simulink model "DroneModelV2"  (R2024a)
settings: Solver=VariableStepAuto  StartTime=0.0  StopTime=7  RelTol=1e-3
values from neighbouring files (symbols this model uses):
  drag_co = torque_Nm / no_rot^2    (= 9.75332775919e-12)    [QuadcopterAttributes.m]
  g = 9.81    [StateSpace.m]
  KV_rating = 2800    [QuadcopterAttributes.m]
  lift_co = thrust_N / no_rot^2    (= 5.88883004597e-10)    [QuadcopterAttributes.m]
  m = 0.5    [StateSpace.m]
  r = 0.25    [StateSpace.m]
undefined symbols (not defined in the file or in its folder): I_p
libraries: simulink x2, shared6dof x1
settings Model: Creator=Henrik  LastModifiedBy=Henrik

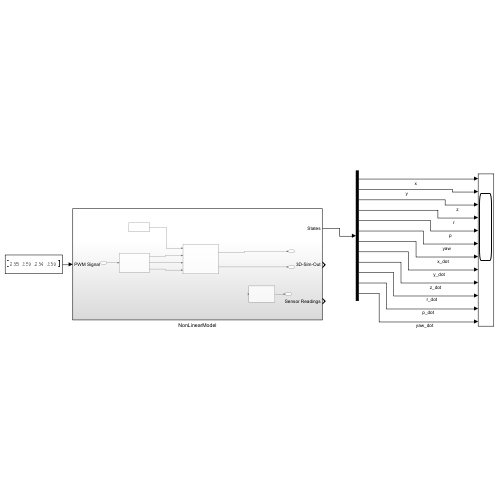
[thumbnail: Simulink's stored preview of the top-level diagram]
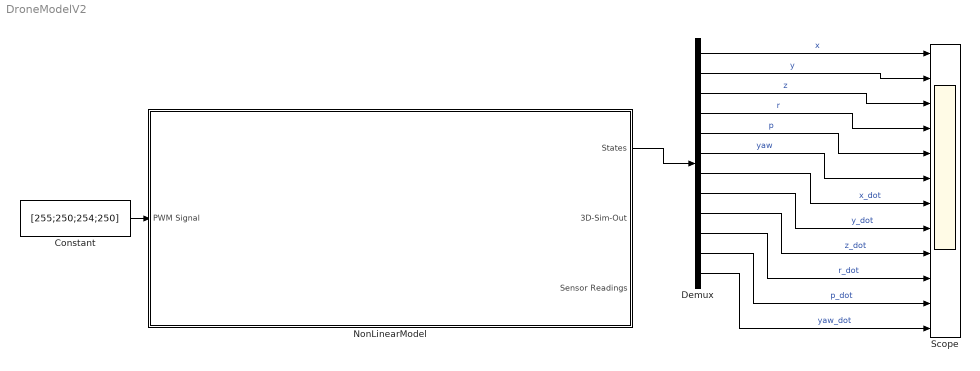
== system DroneModelV2 ==
  Constant : Constant  Value=[255;250;254;250]
  Demux : Demux  Outputs=12
  NonLinearModel : Subsystem
  Scope : Scope  NumInputPorts=12
  wires:
  Constant/1 -> NonLinearModel/1(PWM Signal)
  NonLinearModel/1(States) -> Demux/1
  Demux/1 -> Scope/1  "x"
  Demux/2 -> Scope/2  "y"
  Demux/3 -> Scope/3  "z"
  Demux/4 -> Scope/4  "r"
  Demux/5 -> Scope/5  "p"
  Demux/6 -> Scope/6  "yaw"
  Demux/7 -> Scope/7  "x_dot"
  Demux/8 -> Scope/8  "y_dot"
  Demux/9 -> Scope/9  "z_dot"
  Demux/10 -> Scope/10  "r_dot"
  Demux/11 -> Scope/11  "p_dot"
  Demux/12 -> Scope/12  "yaw_dot"

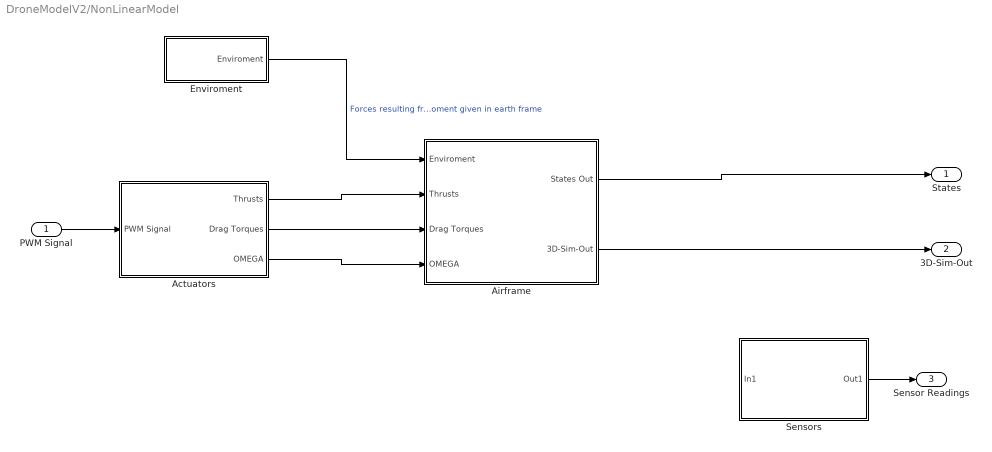
== system DroneModelV2/NonLinearModel ==
  PWM Signal : Inport
  Actuators : Subsystem
  Airframe : Subsystem
  Enviroment : Subsystem
  Sensors : Subsystem
  States : Outport
  3D-Sim-Out : Outport  Port=2
  Sensor Readings : Outport  Port=3
  wires:
  PWM Signal/1 -> Actuators/1(PWM Signal)
  Airframe/1(States Out) -> States/1
  Enviroment/1(Enviroment) -> Airframe/1(Enviroment)  "Forces resulting from enviroment given in earth frame"
  Actuators/1(Thrusts) -> Airframe/2(Thrusts)
  Airframe/2(3D-Sim-Out) -> 3D-Sim-Out/1
  Actuators/2(Drag Torques) -> Airframe/3(Drag Torques)
  Actuators/3(OMEGA) -> Airframe/4(OMEGA)
  Sensors/1(Out1) -> Sensor Readings/1

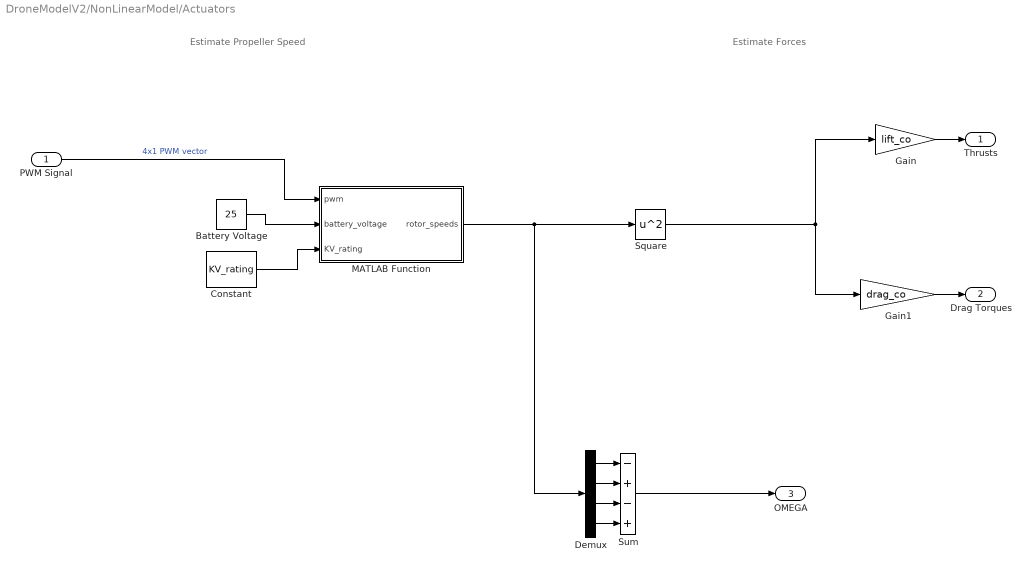
== system DroneModelV2/NonLinearModel/Actuators ==
  note: Estimate Forces
  note: Estimate Propeller Speed
  PWM Signal : Inport
  Battery Voltage : Constant  Value=25
  Constant : Constant  Value=KV_rating
  Demux : Demux
  Gain : Gain  Gain=lift_co
  Gain1 : Gain  Gain=drag_co
  MATLAB Function : MATLAB Function  TreatAsAtomicUnit=on
  Square : Math  Operator=square
  Sum : Sum  Inputs=-+-+
  Thrusts : Outport
  Drag Torques : Outport  Port=2
  OMEGA : Outport  Port=3
  wires:
  Constant/1 -> MATLAB Function/3(KV_rating)
  Battery Voltage/1 -> MATLAB Function/2(battery_voltage)
  PWM Signal/1 -> MATLAB Function/1(pwm)  "4x1 PWM vector"
  MATLAB Function/1(rotor_speeds) -> Square/1, Demux/1
  Gain/1 -> Thrusts/1
  Square/1 -> Gain/1, Gain1/1
  Gain1/1 -> Drag Torques/1
  Demux/1 -> Sum/1
  Demux/2 -> Sum/2
  Demux/3 -> Sum/3
  Demux/4 -> Sum/4
  Sum/1 -> OMEGA/1

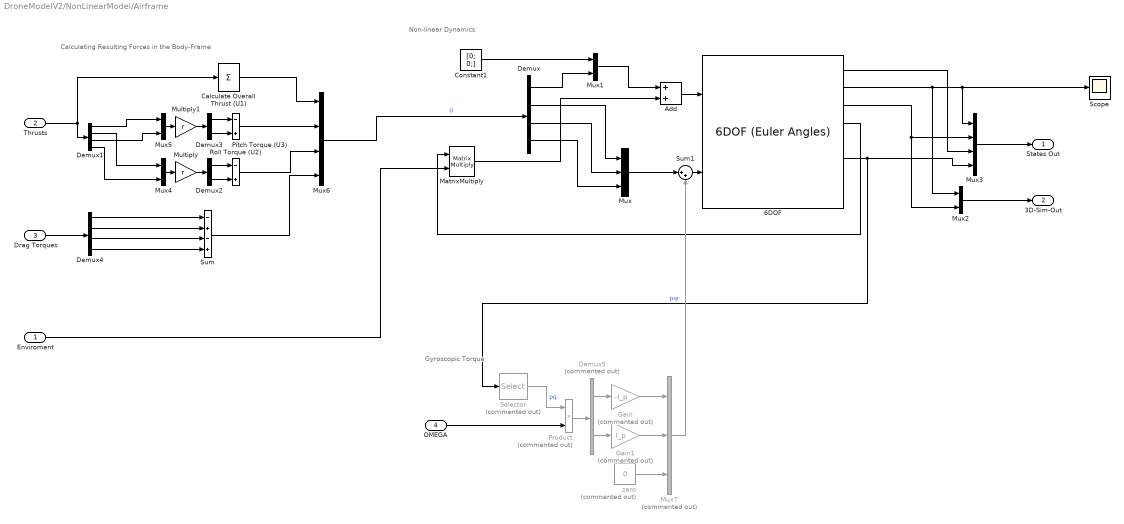
== system DroneModelV2/NonLinearModel/Airframe ==
  note: Gyroscopic Torque
  note: Non-linear Dynamics
  note: Calculating Resulting Forces in the Body-Frame
  Enviroment : Inport
  Thrusts : Inport  Port=2
  Drag Torques : Inport  Port=3
  OMEGA : Inport  Port=4
  "6DOF " : shared6dof/6DOF (Euler Angles)  units=Metric (MKS)  mtype=Fixed  rep=Quaternion  xme_0=[0 0 0]  Vm_0=[0 0 0]  eul_0=[0 0 0]  pm_0=[0 0 0]  mass_0=m  mass_e=0.5  mass_f=2.0  inertia=Inertia_Mat  inertia_e=eye(3)  inertia_f=2*eye(3)  k_quat=1.0  vre_flag=on  abi_flag=off  aMode=0  xme_statename=''  Vm_statename=''  eul_statename=''  quat_statename=''  pm_statename=''  mass_statename=''
      settings: LibrarySourceBlock=aerolib6dof2/6DOF (Quaternion)
  Add : Sum
  "Calculate Overall Thrust (U1) " : Sum  Inputs=+
  Constant1 : Constant  Value=[0; 0;]
  Demux : Demux
  Demux1 : Demux
  Demux2 : Demux  Outputs=2
  Demux3 : Demux  Outputs=2
  Demux4 : Demux
  Demux5 : Demux  Commented=on  Outputs=2
  Gain : Gain  Commented=on  Gain=-I_p
  Gain1 : Gain  Commented=on  Gain=I_p
  MatrixMultiply : Product  Multiplication=Matrix(*)
  Multiply : Gain  Gain=r
  Multiply1 : Gain  Gain=r
  Mux : Mux  Inputs=3
  Mux{1..2,4..5} (4 alike) : Mux  Inputs=2
  Mux3 : Mux
  Mux6 : Mux
  Mux7 : Mux  Commented=on  Inputs=3
  Pitch Torque (U3) : Sum  Inputs=-+
  Product : Product  Commented=on
  Roll Torque (U2) : Sum  Inputs=-+
  Scope : Scope
  Selector : Selector  Commented=on  InputPortWidth=3  IndexOptions=Index vector (dialog)  Indices=[1 2]  OutputSizes=1
  Sum : Sum  Inputs=-+-+
  Sum1 : Sum  Inputs=|++
  zero : Constant  Commented=on  Value=0
  States Out : Outport
  3D-Sim-Out : Outport  Port=2
  wires:
  Demux/2 -> Mux/1
  Demux/3 -> Mux/2
  Demux/4 -> Mux/3
  Enviroment/1 -> MatrixMultiply/2
  "6DOF "/4 -> MatrixMultiply/1
  Add/1 -> "6DOF "/1
  MatrixMultiply/1 -> Add/2
  "6DOF "/2 -> Mux2/1, Mux3/1, Scope/1
  Demux/1 -> Mux1/2
  Constant1/1 -> Mux1/1
  Mux1/1 -> Add/1
  Mux2/1 -> 3D-Sim-Out/1
  "6DOF "/3 -> Mux3/2, Mux2/2
  "6DOF "/1 -> Mux3/3
  "6DOF "/6 -> Mux3/4, Selector/1  "pqr"
  Mux3/1 -> States Out/1
  Thrusts/1 -> "Calculate Overall Thrust (U1) "/1, Demux1/1
  Demux1/4 -> Mux4/2
  Demux1/2 -> Mux4/1
  Mux4/1 -> Multiply/1
  Multiply/1 -> Demux2/1
  Demux2/1 -> Roll Torque (U2)/1
  Demux2/2 -> Roll Torque (U2)/2
  Mux5/1 -> Multiply1/1
  Demux1/1 -> Mux5/1
  Multiply1/1 -> Demux3/1
  Demux3/2 -> Pitch Torque (U3)/2
  Demux3/1 -> Pitch Torque (U3)/1
  Demux1/3 -> Mux5/2
  "Calculate Overall Thrust (U1) "/1 -> Mux6/1
  Pitch Torque (U3)/1 -> Mux6/2
  Roll Torque (U2)/1 -> Mux6/3
  Mux6/1 -> Demux/1  "U"
  Drag Torques/1 -> Demux4/1
  Demux4/3 -> Sum/3
  Demux4/4 -> Sum/4
  Demux4/1 -> Sum/1
  Demux4/2 -> Sum/2
  Sum/1 -> Mux6/4
  OMEGA/1 -> Product/2
  Selector/1 -> Product/1  "pq"
  Product/1 -> Demux5/1
  Demux5/1 -> Gain/1
  Demux5/2 -> Gain1/1
  Gain/1 -> Mux7/1
  Gain1/1 -> Mux7/2
  zero/1 -> Mux7/3
  Mux/1 -> Sum1/1
  Mux7/1 -> Sum1/2
  Sum1/1 -> "6DOF "/2

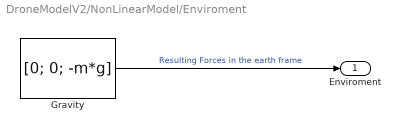
== system DroneModelV2/NonLinearModel/Enviroment ==
  Gravity : Constant  Value=[0; 0; -m*g]
  Enviroment : Outport
  wires:
  Gravity/1 -> Enviroment/1  "Resulting Forces in the earth frame"

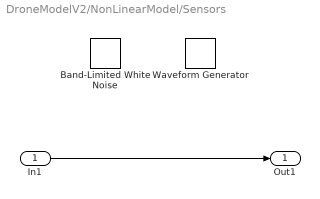
== system DroneModelV2/NonLinearModel/Sensors ==
  In1 : Inport
  Band-Limited White Noise : simulink/Sources/Band-Limited White Noise  Cov=[0.1]  Ts=0.1  seed=[23341]
  Waveform Generator : simulink/Sources/Waveform Generator  OutMin=[]  OutMax=[]  OutDataTypeStr=double  SelectedSignal=1  BlockNames=MultiportSwitch_e3df3653d217406  SampleTime=0.1
  Out1 : Outport
  wires:
  In1/1 -> Out1/1

== matlab function DroneModelV2/NonLinearModel/Actuators/MATLAB Function ==
  data: pwm input; rotor_speeds output; battery_voltage input; KV_rating input
function rotor_speeds = fcn(pwm, battery_voltage, KV_rating)
    
    rotor_speeds = zeros(4,1); % Initialize rotor_speeds
    
    for i = 1:1:4
    
        duty_cycle = pwm(i,1)/255;
        rotor_speeds(i,1) = duty_cycle * battery_voltage * KV_rating;
    
    end

end
